simulink model "TutoAltera"  (R2016a)
settings: Solver=FixedStepDiscrete  SolverMode=SingleTasking  StartTime=0.0  StopTime=4E-6  RelTol=1e-3
InitFcn:
  | %% DSPBuilder Start
  | alt_dspbuilder_update_model(bdroot)
  | %% DSPBuilder End
libraries: allblocks_alteradspbuilder2 x11
settings Model: Creator=souc2303  LastModifiedBy=souc2303

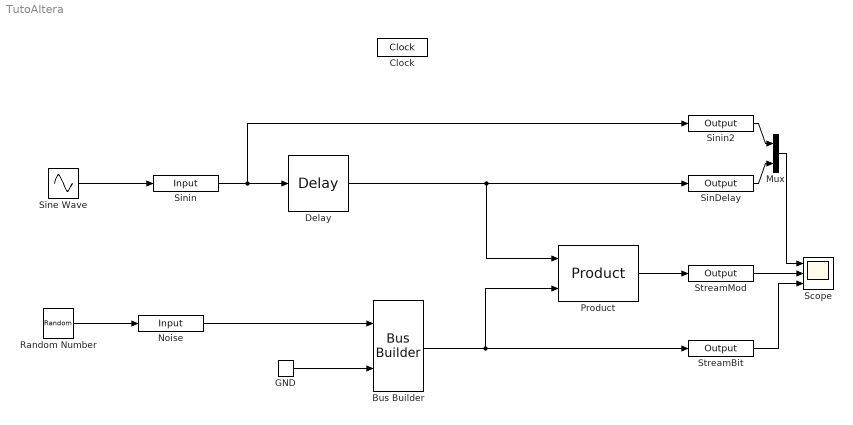
== system TutoAltera ==
  Bus Builder : allblocks_alteradspbuilder2/Bus Builder  BusType=Signed Integer  bwl=2  bwr=1  pipeline_display=0
  Clock : allblocks_alteradspbuilder2/Clock  ClockPeriod=20  ClockPeriodUnit=ns  SampleTime=25E-9  ResetLatency=0  ResetRegisterCascadeDepth=0  SimulationStartCycle=5  PhaseOffset=0  Reset=aclr  ResetType=Active Low  Export=off
  Delay : allblocks_alteradspbuilder2/Delay  pipeline=1  pipeline_display=1  ClockPhase=01  use_ena=off  use_sclr=off  allowFloatingPointOverride=on  logOutputs=off  logFile=U:\DSPBuilder\tb_Singen\Singen_Delay.fixedpointlog  use_init=off  reset_value=1
  GND : allblocks_alteradspbuilder2/GND  SpecifyClock=off
  Mux : Mux  Inputs=2
  Noise : allblocks_alteradspbuilder2/Input  iofile=U:\DSPBuilder\tb_Singen\Singen_Noise.salt  BusType=Single Bit  bwl=2  bwr=0  SpecifyClock=off  PORTTYPE=Input  externalType=Inferred  allowFloatingPointOverride=on  logOutputs=off
  Product : allblocks_alteradspbuilder2/Product  BusType=Inferred  bwl=8  bwr=0  pipeline=0  pipeline_display=0  phase_selection=1  use_ena=off  use_aclr=off  UseLPM=off  UseDedicatedCircuitry=on  allowFloatingPointOverride=on  logOutputs=off  logFile=U:\DSPBuilder\tb_Singen\Singen_Product.fixedpointlog
  Random Number : RandomNumber  SampleTime=25e-9
  Scope : Scope  NumInputPorts=3
  SinDelay : allblocks_alteradspbuilder2/Output  iofile=U:\DSPBuilder\tb_Singen\Singen_SinDelay.capture  BusType=Signed Integer  bwl=16  bwr=0  externalType=Inferred  PORTTYPE=Output  allowFloatingPointOverride=on  logOutputs=off
  Sine Wave : Sin  SineType=Sample based  Amplitude=2^15-1  Samples=80  SampleTime=25E-9
  Sinin : allblocks_alteradspbuilder2/Input  iofile=U:\DSPBuilder\tb_Singen\Singen_Sinin.salt  BusType=Signed Integer  bwl=16  bwr=0  SpecifyClock=off  PORTTYPE=Input  externalType=Inferred  allowFloatingPointOverride=on  logOutputs=off
  Sinin2 : allblocks_alteradspbuilder2/Output  iofile=U:\DSPBuilder\tb_Singen\Singen_Sinin2.capture  BusType=Signed Integer  bwl=16  bwr=0  externalType=Inferred  PORTTYPE=Output  allowFloatingPointOverride=on  logOutputs=off
  StreamBit : allblocks_alteradspbuilder2/Output  iofile=U:\DSPBuilder\tb_Singen\Singen_StreamBit.capture  BusType=Single Bit  bwl=16  bwr=0  externalType=Inferred  PORTTYPE=Output  allowFloatingPointOverride=on  logOutputs=off
  StreamMod : allblocks_alteradspbuilder2/Output  iofile=U:\DSPBuilder\tb_Singen\Singen_StreamMod.capture  BusType=Signed Integer  bwl=19  bwr=0  externalType=Inferred  PORTTYPE=Output  allowFloatingPointOverride=on  logOutputs=off
  wires:
  Sine Wave/1 -> Sinin/1
  Sinin/1 -> Sinin2/1, Delay/1
  Delay/1 -> Product/1, SinDelay/1
  Random Number/1 -> Noise/1
  Noise/1 -> Bus Builder/1
  GND/1 -> Bus Builder/2
  Sinin2/1 -> Mux/1
  SinDelay/1 -> Mux/2
  Product/1 -> StreamMod/1
  Bus Builder/1 -> Product/2, StreamBit/1
  StreamMod/1 -> Scope/2
  Mux/1 -> Scope/1
  StreamBit/1 -> Scope/3
